simulink model "Simulink_Test_Model_Simple"  (R2018a)
settings: Solver=VariableStepAuto  StartTime=0.0  StopTime=10.0  RelTol=1e-3
libraries: simulink x1
settings Model: Creator=user  LastModifiedBy=user

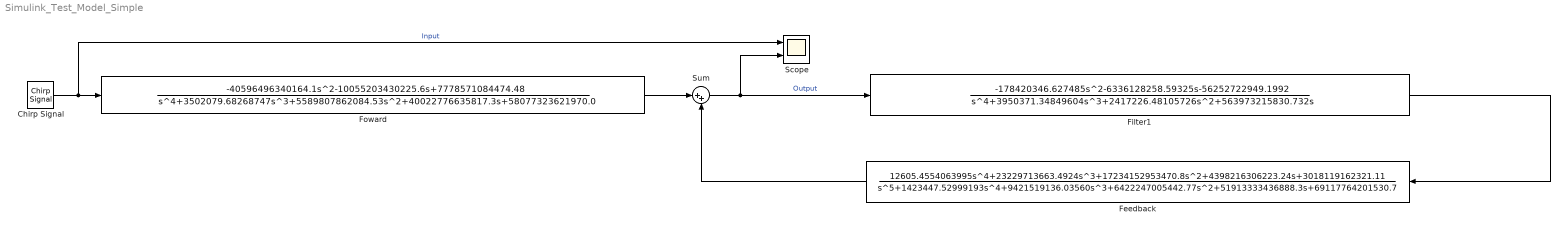
== system Simulink_Test_Model_Simple ==
  Chirp Signal : simulink/Sources/Chirp Signal  f1=20  T=10  f2=80
  Feedback : TransferFcn  Numerator=[12605.4554063995,23229713663.4924,17234152953470.8,4398216306223.24,3018119162321.11]  Denominator=[1,1423447.52999193,9421519136.03560,6422247005442.77,51913333436888.3,69117764201530.7]
  Filter1 : TransferFcn  Numerator=[-178420346.627485 -6336128258.59325 -56252722949.1992]  Denominator=[1 3950371.34849604 2417226.48105726 563973215830.732 0]
  Foward : TransferFcn  Numerator=[-40596496340164.1,-10055203430225.6,7778571084474.48]  Denominator=[1,3502079.68268747,5589807862084.53,40022776635817.3,58077323621970.0]
  Scope : Scope  NumInputPorts=2
  Sum : Sum  Inputs=|++  OutMin=[-100]  OutMax=[100]
  wires:
  Foward/1 -> Sum/1
  Sum/1 -> Filter1/1, Scope/2  "Output"
  Chirp Signal/1 -> Scope/1, Foward/1  "Input"
  Filter1/1 -> Feedback/1
  Feedback/1 -> Sum/2
